simulink model "Neutron_e"  (Simulink 7.9)
settings: Solver=ode45  StartTime=0.0  StopTime=10.0  RelTol=1e-3
values from neighbouring files (symbols this model uses):
  a = -1.0    (= -1)    [parameters.m]
  b = -2.0    (= -2)    [parameters.m]
  c = 0.23    [parameters.m]
  Ta = 0.38    [parameters.m]
  Tr = 0.04    [parameters.m]
settings Model: Creator=dede  LastModifiedBy=dede

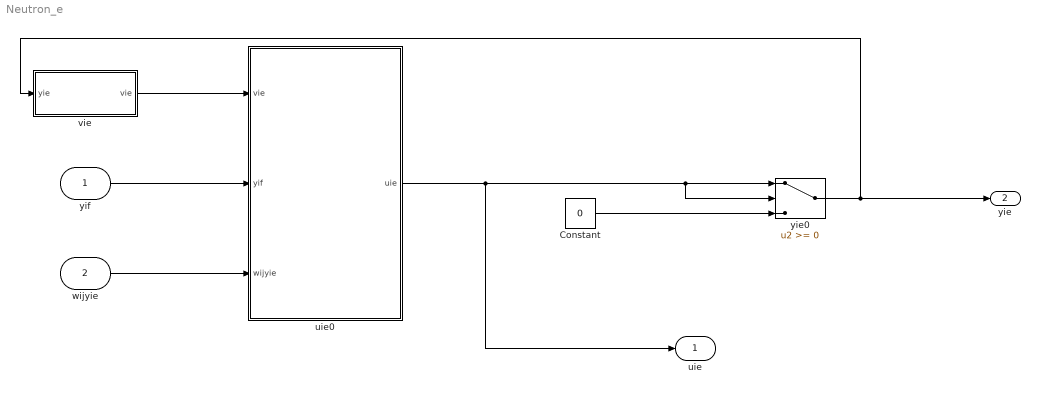
== system Neutron_e ==
  yif : Inport
  wijyie : Inport  Port=2
  Constant : Constant  Value=0
  uie0 : Subsystem
  vie : Subsystem
  yie0 : Switch
  uie : Outport
  yie : Outport  Port=2
  wires:
  vie/1(vie) -> uie0/1(vie)
  yif/1 -> uie0/2(yif)
  wijyie/1 -> uie0/3(wijyie)
  Constant/1 -> yie0/3
  uie0/1(uie) -> yie0/1, yie0/2, uie/1
  yie0/1 -> vie/1(yie), yie/1

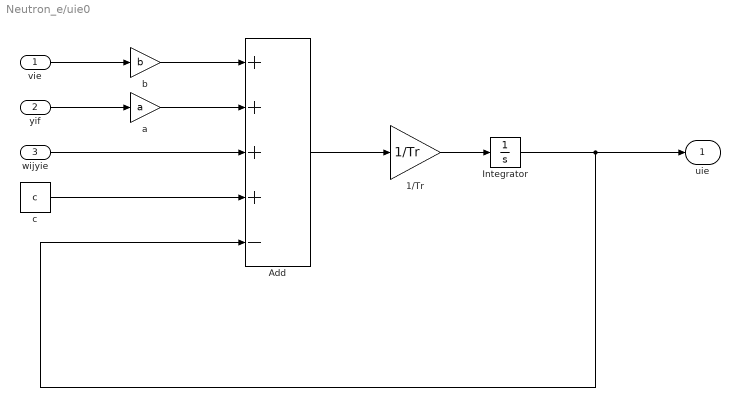
== system Neutron_e/uie0 ==
  vie : Inport
  yif : Inport  Port=2
  wijyie : Inport  Port=3
  1/Tr : Gain  Gain=1/Tr
  Add : Sum  Inputs=++++-
  Integrator : Integrator
  a : Gain  Gain=a
  b : Gain  Gain=b
  c : Constant  Value=c
  uie : Outport
  wires:
  vie/1 -> b/1
  b/1 -> Add/1
  yif/1 -> a/1
  a/1 -> Add/2
  wijyie/1 -> Add/3
  c/1 -> Add/4
  Add/1 -> 1/Tr/1
  1/Tr/1 -> Integrator/1
  Integrator/1 -> Add/5, uie/1

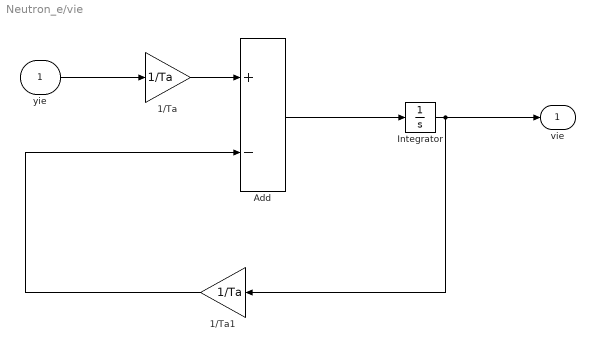
== system Neutron_e/vie ==
  yie : Inport
  1/Ta : Gain  Gain=1/Ta
  1/Ta1 : Gain  Gain=1/Ta
  Add : Sum  Inputs=+-
  Integrator : Integrator
  vie : Outport
  wires:
  yie/1 -> 1/Ta/1
  1/Ta/1 -> Add/1
  Add/1 -> Integrator/1
  Integrator/1 -> 1/Ta1/1, vie/1
  1/Ta1/1 -> Add/2
